simulink model "modelo_EHA"  (R2014b)
settings: Solver=ode45  StartTime=0  StopTime=2  RelTol=1e-3
undefined symbols (not defined in the file or in its folder): D0, D1, D2, D3, degrau, N0
libraries: powerlib x3, simulink x2, electricdrivelib x1, AC7DriveInternalModels x1, dspstat3 x1
settings Model: Creator=Joao  LastModifiedBy=JPSOLIV
settings DataIOCC: LimitDataPoints=off

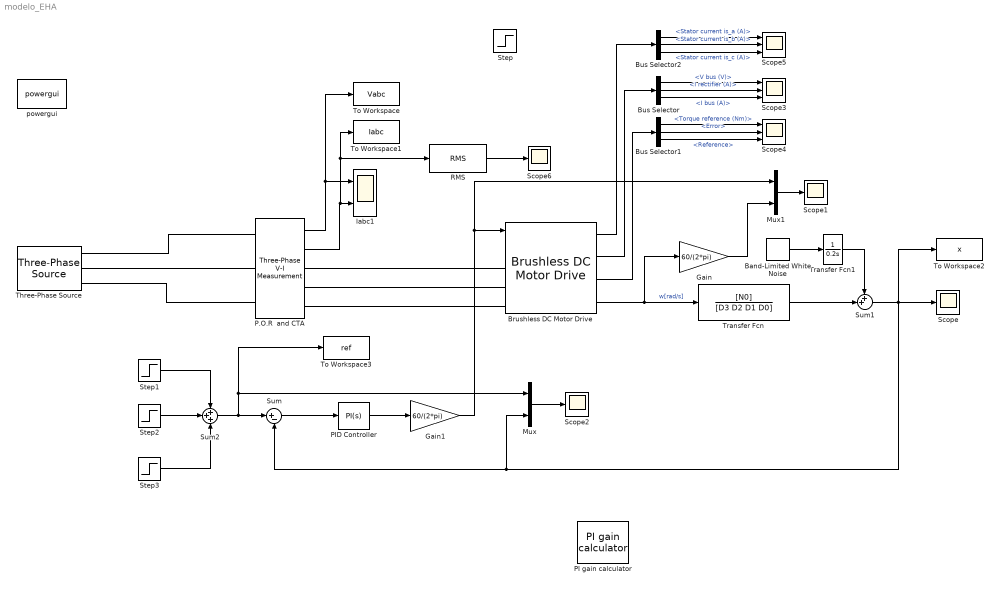
== system modelo_EHA ==
  Band-Limited White Noise : simulink/Sources/Band-Limited White Noise  Cov=[0.00003*0]  Ts=0.15  seed=[233410]
  Brushless DC Motor Drive : electricdrivelib/AC drives/Brushless DC Motor Drive  showMaskWarnings=on  AverageValue=off  MechanicalLoad=Torque Tm  driveType=AC7  outputBusMode=Multiple output buses
  Bus Selector : BusSelector  OutputSignals=V bus (V),I rectifier (A),I bus (A)
  Bus Selector1 : BusSelector  OutputSignals=Torque reference (Nm),Error,Reference
  Bus Selector2 : BusSelector  OutputSignals=Stator current is_a (A),Stator current is_b (A),Stator current is_c (A)
  Gain : Gain  Gain=60/(2*pi)
  Gain1 : Gain  Gain=60/(2*pi)
  Iabc1 : Scope  NumInputPorts=2
      settings: TimeRange=0.005  YMin=-200~-0.8  YMax=200~0.8  SaveName=vac1  SampleTime=10e-6
  Mux : Mux  Inputs=2
  Mux1 : Mux  Inputs=2
  P.O.R  and CTA : powerlib/Measurements/Three-Phase V-I Measurement  VoltageMeasurement=phase-to-ground  SetLabelV=off  LabelV=Vabc  Vpu=off  VpuLL=off  CurrentMeasurement=yes  SetLabelI=off  LabelI=Iabc  Ipu=off  Pbase=100e6  Vbase=500e3  OutputType=Complex  PhasorSimulation=off  PSBequivalent=0
  PI gain calculator : AC7DriveInternalModels/PI gain calculator  mec=[0.089 0.005 4]  specs=on  ele=[0.2 8.5e-3]  lam=0.175  open_loop=off  zeta=0.99  Trd=0.13/5  check=off
  PID Controller : simulink/Continuous/PID Controller  Controller=PI  TimeDomain=Continuous-time  SampleTime=-1  IntegratorMethod=Forward Euler  FilterMethod=Forward Euler  Form=Parallel  P=100  I=1600  D=0  N=100  InitialConditionSource=internal  InitialConditionForIntegrator=0  InitialConditionForFilter=0  ExternalReset=none  LimitOutput=off  UpperSaturationLimit=inf  LowerSaturationLimit=-inf  LinearizeAsGain=on  AntiWindupMode=none  Kb=1  TrackingMode=off  Kt=1  PParamMin=[]  PParamMax=[]  IParamMin=[]  IParamMax=[]  DParamMin=[]  DParamMax=[]  NParamMin=[]  NParamMax=[]  KbParamMin=[]  KbParamMax=[]  KtParamMin=[]  KtParamMax=[]  POutMin=[]  POutMax=[]  IOutMin=[]  IOutMax=[]  DOutMin=[]  DOutMax=[]  NOutMin=[]  NOutMax=[]  KbOutMin=[]  KbOutMax=[]  KtOutMin=[]  KtOutMax=[]  IntegratorOutMin=[]  IntegratorOutMax=[]  FilterOutMin=[]  FilterOutMax=[]  SumOutMin=[]  SumOutMax=[]  SumI1OutMin=[]  SumI1OutMax=[]  SumI2OutMin=[]  SumI2OutMax=[]  SumI3OutMin=[]  SumI3OutMax=[]  SumDOutMin=[]  SumDOutMax=[]  SaturationOutMin=[]  SaturationOutMax=[]  IntegratorContinuousStateAttributes=''  IntegratorStateMustResolveToSignalObject=off  IntegratorRTWStateStorageClass=Auto  FilterContinuousStateAttributes=''  FilterStateMustResolveToSignalObject=off  FilterRTWStateStorageClass=Auto  DifferentiatorICPrevScaledInput=0  DifferentiatorOutMin=[]  DifferentiatorOutMax=[]  UseFilter=on
  RMS : dspstat3/RMS  run=off  reset_popup=None  InputProcessing=Columns as channels (frame based)  directionMode=Each column  dimension=1  treatSBRowAsCol=on
  Scope{,1..2,6} (4 alike) : Scope
      Scope settings: YMin=-1e-05  YMax=6e-05
      Scope1 settings: YMin=-30  YMax=30
      Scope2 settings: YMin=-0.01  YMax=0.02  SaveName=ScopeData2
      Scope6 settings: YMin=0  YMax=90000  SaveName=ScopeData6
  Scope3 : Scope  NumInputPorts=3
      settings: YMin=0~0~-100  YMax=300~60~100  SaveName=ScopeData3
  Scope4 : Scope  NumInputPorts=3
      settings: YMin=0~0~-40  YMax=150~30~40  SaveName=ScopeData4
  Scope5 : Scope  NumInputPorts=3
      settings: YMin=0~0~-40  YMax=150~30~40  SaveName=ScopeData5
  Step : Step  Time=0.5  After=1685*2  SampleTime=0
  Step1 : Step  Time=0  Before=degrau  After=degrau  SampleTime=0
  Step2 : Step  After=-2*degrau  SampleTime=0
  Step3 : Step  Time=2.1  After=degrau  SampleTime=0
  Sum : Sum  Inputs=|+-
  Sum1 : Sum  Inputs=++|
  Sum2 : Sum  Inputs=+++
  Three-Phase Source : powerlib/Electrical Sources/Three-Phase Source  Voltage=115*sqrt(3)  PhaseAngle=0  Frequency=400  InternalConnection=Yg  SpecifyImpedance=off  Resistance=1e-2  Inductance=10e-4  ShortCircuitLevel=100e6  BaseVoltage=25e3  XRratio=7  BusType=swing  Pref=0  Qref=0  Qmin=-inf  Qmax=inf
  To Workspace : ToWorkspace  VariableName=Vabc  SaveFormat=Structure With Time  SampleTime=-1
  To Workspace1 : ToWorkspace  VariableName=Iabc  SaveFormat=Structure With Time  SampleTime=-1
  To Workspace2 : ToWorkspace  VariableName=x  SaveFormat=Structure With Time  SampleTime=-1
  To Workspace3 : ToWorkspace  VariableName=ref  SaveFormat=Structure With Time  SampleTime=-1
  Transfer Fcn : TransferFcn  Numerator=[N0]  Denominator=[D3 D2 D1 D0]
  Transfer Fcn1 : TransferFcn  Denominator=[0.2 0]
  powergui : powerlib/powergui  Priority=1  SimulationMode=Discrete  SolverType=Tustin  SampleTime=5e-6  frequency=60  SPID=off  DisableSnubberDevices=off  DisableRonSwitches=off  DisableVfSwitches=off  SwTol=0  DisplayEquations=off  Interpol=off  methode=off  Ts=0  frequencyindice=0  Pbase=100e6  ErrMax=1e-4  Iterations=50  UnitsV=kV  UnitsW=MW  FunctionMessages=off  echomessages=off  HookPort=off  EnableUseOfTLC=off  x0status=blocks  RestoreLinks=warning  ResistiveCurrentMeasurement=off  Frange=[0:2:500]  Ylog=off  Xlog=on  ShowGrid=off  save=off  variable=ZData  structure=0  ZoomFFT=off  StartTime=0.0  cycles=1  DisplayStyle=1  fundamental=60  FreqAxis=off  MaxFrequency=1000  frequencyindicesteady=1  RmsSteady=1  display=off
  wires:
  Brushless DC Motor Drive/4 -> Gain/1, Transfer Fcn/1  "w[rad/s]"
  P.O.R  and CTA/1 -> To Workspace/1, Iabc1/1
  P.O.R  and CTA/2 -> RMS/1, To Workspace1/1, Iabc1/2
  Gain/1 -> Mux1/2
  Step1/1 -> Sum2/1
  Mux/1 -> Scope2/1
  PID Controller/1 -> Gain1/1
  Mux1/1 -> Scope1/1
  Gain1/1 -> Brushless DC Motor Drive/1, Mux1/1
  Transfer Fcn/1 -> Sum1/2
  Sum1/1 -> To Workspace2/1, Mux/2, Sum/2, Scope/1
  Sum2/1 -> To Workspace3/1, Mux/1, Sum/1
  Step2/1 -> Sum2/2
  Step3/1 -> Sum2/3
  Band-Limited White Noise/1 -> Transfer Fcn1/1
  Transfer Fcn1/1 -> Sum1/1
  Brushless DC Motor Drive/2 -> Bus Selector/1
  Bus Selector/1 -> Scope3/1  "<V bus (V)>"
  Bus Selector/2 -> Scope3/2  "<I rectifier (A)>"
  Bus Selector/3 -> Scope3/3  "<I bus (A)>"
  Brushless DC Motor Drive/3 -> Bus Selector1/1
  Bus Selector1/1 -> Scope4/1  "<Torque reference (Nm)>"
  Bus Selector1/2 -> Scope4/2  "<Error>"
  Bus Selector1/3 -> Scope4/3  "<Reference>"
  Brushless DC Motor Drive/1 -> Bus Selector2/1
  Bus Selector2/1 -> Scope5/1  "<Stator current is_a (A)>"
  Bus Selector2/2 -> Scope5/2  "<Stator current is_b (A)>"
  Bus Selector2/3 -> Scope5/3  "<Stator current is_c (A)>"
  RMS/1 -> Scope6/1
  Sum/1 -> PID Controller/1
  connections:
  Brushless DC Motor Drive/LConn2 -- P.O.R  and CTA/RConn2
  Brushless DC Motor Drive/LConn1 -- P.O.R  and CTA/RConn1
  Brushless DC Motor Drive/LConn3 -- P.O.R  and CTA/RConn3
  Three-Phase Source/RConn2 -- P.O.R  and CTA/LConn2
  Three-Phase Source/RConn1 -- P.O.R  and CTA/LConn1
  Three-Phase Source/RConn3 -- P.O.R  and CTA/LConn3
